simulink model "Subtractor_4BIT"  (R2018a)
settings: Solver=VariableStepAuto  StartTime=0.0  StopTime=10.0  RelTol=1e-3
settings Model: Creator=midog  LastModifiedBy=midog

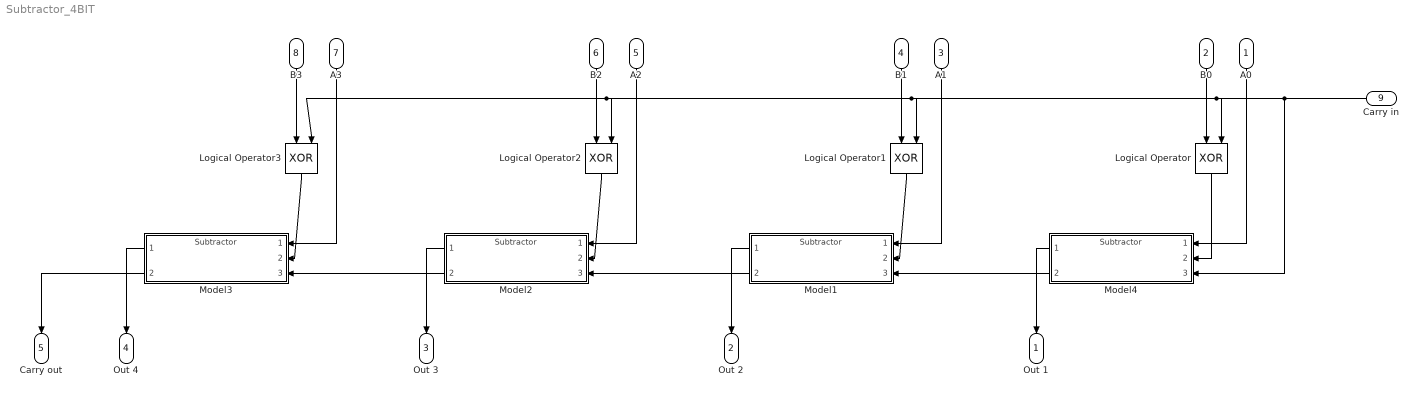
== system Subtractor_4BIT ==
  A0 : Inport
  B0 : Inport  Port=2
  A1 : Inport  Port=3
  B1 : Inport  Port=4
  A2 : Inport  Port=5
  B2 : Inport  Port=6
  A3 : Inport  Port=7
  B3 : Inport  Port=8
  Carry in : Inport  Port=9
  Logical Operator{,1..3} (4 alike) : Logic  Operator=XOR  IconShape=distinctive  AllPortsSameDT=off  OutDataTypeStr=boolean
  Model{1..4} (4 alike) : ModelReference  ModelNameDialog=Subtractor  SimulationMode=Normal  ModelReferenceVersion=1.1
  Out 1 : Outport
  Out 2 : Outport  Port=2
  Out 3 : Outport  Port=3
  Out 4 : Outport  Port=4
  Carry out : Outport  Port=5
  wires:
  Carry in/1 -> Model4/3, Logical Operator3/2, Logical Operator2/2, Logical Operator1/2, Logical Operator/2
  B3/1 -> Logical Operator3/1
  Logical Operator/1 -> Model4/2
  A3/1 -> Model3/1
  Model2/2 -> Model3/3
  A2/1 -> Model2/1
  B2/1 -> Logical Operator2/1
  Logical Operator2/1 -> Model2/2
  Model1/2 -> Model2/3
  Model4/1 -> Out 1/1
  Model1/1 -> Out 2/1
  A1/1 -> Model1/1
  B0/1 -> Logical Operator/1
  A0/1 -> Model4/1
  Model2/1 -> Out 3/1
  Model3/1 -> Out 4/1
  B1/1 -> Logical Operator1/1
  Model3/2 -> Carry out/1
  Model4/2 -> Model1/3
  Logical Operator3/1 -> Model3/2
  Logical Operator1/1 -> Model1/2
